simulink model "Fact"  (R2021a)
settings: Solver=FixedStepDiscrete  StartTime=0.0  StopTime=10.0  RelTol=1e-3  EnableMultiTasking=on
settings Model: Creator=Osman  LastModifiedBy=Osman
settings DataIOCC: ReturnWorkspaceOutputs=off
settings OptimizationCC: DefaultParameterBehavior=Inlined  InlineInvariantSignals=on  EnableMemcpy=off  LifeSpan=1  EfficientTunableParamExpr=on
settings DebuggingCC: UnderspecifiedInitializationDetection=Classic  MergeDetectMultiDrivingBlocksExec=none  SFMachineParentedDataDiag=warning  ArithmeticOperatorsInVariantConditions=warning
settings ModelReferenceCC: PropagateSignalLabelsOutOfModel=off
settings SFSimCC: MATLABDynamicMemAlloc=off  CustomCodeUndefinedFunction=UseInterfaceOnly
settings RTWCC: SystemTargetFile=ert.tlc  GenCodeOnly=on  TemplateMakefile=ert_default_tmf  GenerateReport=on  IncludeHyperlinkInReport=on  LaunchReport=on  GenerateTraceInfo=on  GenerateTraceReport=on  GenerateTraceReportSl=on  GenerateTraceReportSf=on  GenerateTraceReportEml=on
settings CodeAppCC: ForceParamTrailComments=on  IgnoreCustomStorageClasses=off  OperatorAnnotations=on  SimulinkDataObjDesc=on  SFDataObjDesc=on  MATLABFcnDesc=on  InsertBlockDesc=on  StateflowObjectComments=on  MATLABSourceComments=on
settings ERTTargetCC: MultiwordLength=2048  GenerateSampleERTMain=on  InlinedParameterPlacement=NonHierarchical  ERTCustomFileTemplate=example_file_process.tlc

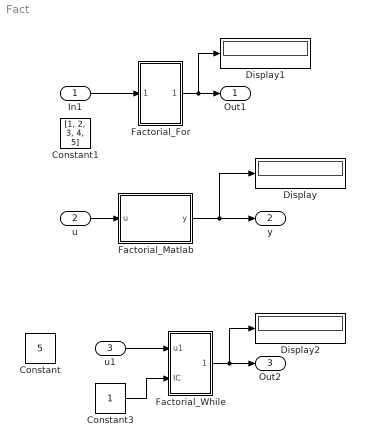
== system Fact ==
  In1 : Inport  PortDimensions=5
  u : Inport  Port=2  OutDataTypeStr=uint32
  u1 : Inport  Port=3  OutDataTypeStr=uint32
  Constant : Constant  Value=5  OutDataTypeStr=uint32
  Constant1 : Constant  Value=[1, 2, 3, 4, 5]  OutDataTypeStr=uint32
  Constant3 : Constant  OutDataTypeStr=uint32
  Display : Display
  Display1 : Display
  Display2 : Display
  Factorial_For : Subsystem  TreatAsAtomicUnit=on  RTWFcnName=Fac_For
      settings: RTWFcnNameOpts=User specified
  Factorial_Matlab : MATLAB Function  TreatAsAtomicUnit=on  RTWFcnName=Fac_Matlab
  Factorial_While : Subsystem  TreatAsAtomicUnit=on  RTWFcnName=Fac_While
      settings: RTWFcnNameOpts=User specified
  Out1 : Outport
  y : Outport  Port=2
  Out2 : Outport  Port=3
  wires:
  Factorial_For/1(Out1) -> Display1/1, Out1/1
  Factorial_Matlab/1(y) -> y/1, Display/1
  In1/1 -> Factorial_For/1(In1)
  u/1 -> Factorial_Matlab/1(u)
  Constant3/1 -> Factorial_While/2(IC)
  Factorial_While/1(Out1) -> Display2/1, Out2/1
  u1/1 -> Factorial_While/1(u1)

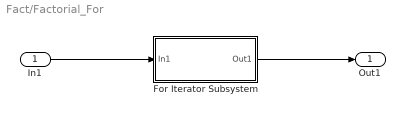
== system Fact/Factorial_For ==
  In1 : Inport  PortDimensions=5
  For Iterator Subsystem : Subsystem  TreatAsAtomicUnit=on
  Out1 : Outport
  wires:
  For Iterator Subsystem/1(Out1) -> Out1/1
  In1/1 -> For Iterator Subsystem/1(In1)

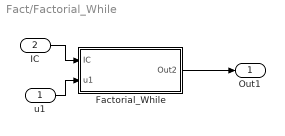
== system Fact/Factorial_While ==
  u1 : Inport  OutDataTypeStr=uint32
  IC : Inport  Port=2
  Factorial_While : Subsystem  TreatAsAtomicUnit=on
  Out1 : Outport
  wires:
  u1/1 -> Factorial_While/2(u1)
  IC/1 -> Factorial_While/1(IC)
  Factorial_While/1(Out2) -> Out1/1

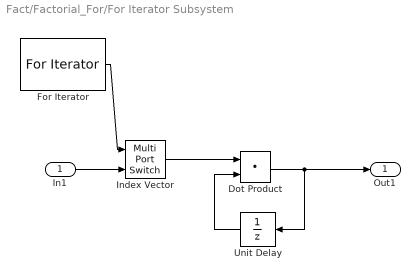
== system Fact/Factorial_For/For Iterator Subsystem ==
  In1 : Inport
  Dot Product : DotProduct  OutDataTypeStr=uint32  InputSameDT=on
  For Iterator : ForIterator  IndexMode=Zero-based
  Index Vector : MultiPortSwitch  DataPortOrder=Zero-based contiguous  Inputs=1  zeroidx=on  OutDataTypeStr=uint32
  Unit Delay : UnitDelay  InitialCondition=1  SampleTime=-1  HasFrameUpgradeWarning=on
  Out1 : Outport
  wires:
  For Iterator/1 -> Index Vector/1
  In1/1 -> Index Vector/2
  Index Vector/1 -> Dot Product/1
  Dot Product/1 -> Unit Delay/1, Out1/1
  Unit Delay/1 -> Dot Product/2

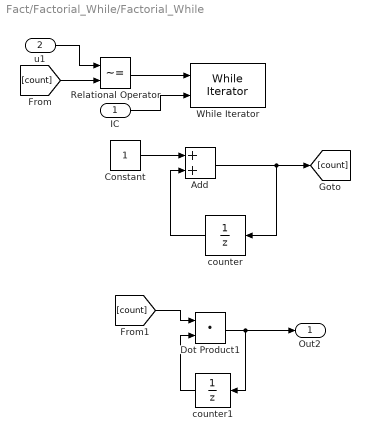
== system Fact/Factorial_While/Factorial_While ==
  IC : Inport
  u1 : Inport  Port=2
  Add : Sum
  Constant : Constant
  Dot Product1 : DotProduct  InputSameDT=on  OutDataTypeStr=Inherit: Inherit via internal rule
  Relational Operator : RelationalOperator  Operator=~=  OutDataTypeStr=boolean  RndMeth=Simplest
  While Iterator : WhileIterator  MaxIters=50
  counter : UnitDelay  SampleTime=-1  HasFrameUpgradeWarning=on
  counter1 : UnitDelay  InitialCondition=1  SampleTime=-1  HasFrameUpgradeWarning=on
  Out2 : Outport
  wires:
  IC/1 -> While Iterator/2
  counter1/1 -> Dot Product1/2
  Dot Product1/1 -> Out2/1, counter1/1
  [count] -> Dot Product1/1
  [count] -> Relational Operator/2
  u1/1 -> Relational Operator/1
  Relational Operator/1 -> While Iterator/1
  Add/1 -> [count], counter/1
  counter/1 -> Add/2
  Constant/1 -> Add/1

== matlab function Fact/Factorial_Matlab ==
  data: u input; y output
function y = fcn(u)
y = uint32(1);
while u > 0
    y = y .* u;
    u = u - 1;
end
